simulink model "AM_signal"  (R2019b)
settings: Solver=VariableStepAuto  StartTime=0.0  StopTime=10.0  RelTol=1e-3
libraries: commchan3 x1, dspsnks4 x1, commanapbnd3 x1
settings Model: Creator=Kai  LastModifiedBy=Kai

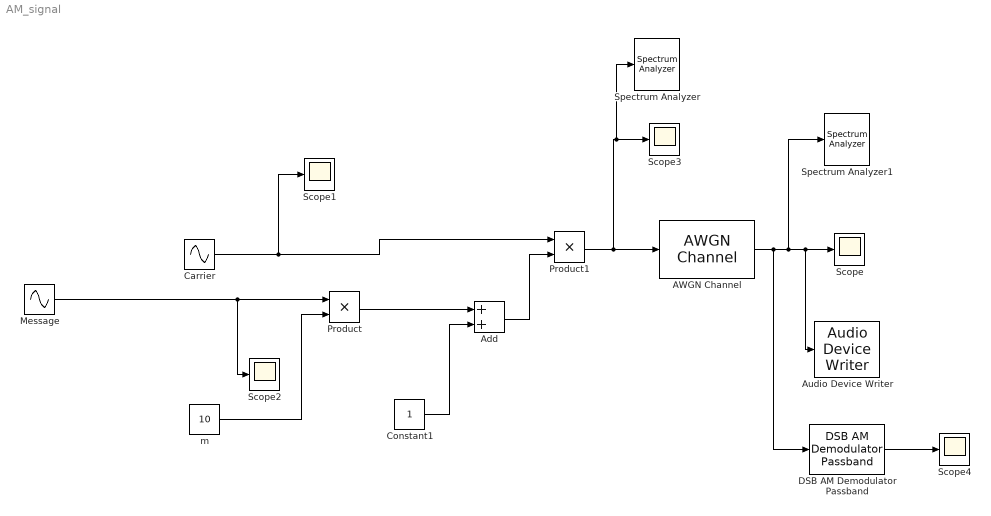
== system AM_signal ==
  AWGN Channel : commchan3/AWGN Channel  InputProcessing=Columns as channels (frame based)  seed=67  noiseMode="Signal to noise ratio  (SNR)"  EbNodB=10  EsNodB=10  SNRdB=3  bitsPerSym=1  Ps=1  Tsym=1  variance=1
      settings: SourceProductName=Communications Toolbox
  Add : Sum
  Audio Device Writer : dspsnks4/Audio Device Writer  Driver=DirectSound  Device=Default  InheritSampleRate=on  SampleRate=44100  BitDepth=16-bit integer  BufferSize=4096  NumBuffers=10  DefaultOutputChannelMapping=on  OutputChannelMapping=1:2  OutputNumUnderrunSamples=off  DriverIdx=1  DeviceWarnFlag=''
  Carrier : Sin  Frequency=2*pi*25  SampleTime=1/50000
  Constant1 : Constant
  DSB AM Demodulator Passband : commanapbnd3/DSB AM Demodulator Passband  Fc=300  Ph=0  method=Butterworth  n=4  cf=300  Rp=0.1  Rs=50  Offset=1
      settings: SourceProductName=Communications Toolbox  SourceProductBaseCode=CM
  "Message " : Sin  Frequency=2*pi  SampleTime=1/50000
  Product : Product
  Product1 : Product
  Scope{,1..4} (5 alike) : Scope
  Spectrum Analyzer : SpectrumAnalyzer
  Spectrum Analyzer1 : SpectrumAnalyzer
  m : Constant  Value=10
  wires:
  "Message "/1 -> Scope2/1, Product/1
  m/1 -> Product/2
  Carrier/1 -> Scope1/1, Product1/1
  Product/1 -> Add/1
  Constant1/1 -> Add/2
  Add/1 -> Product1/2
  AWGN Channel/1 -> DSB AM Demodulator Passband/1, Spectrum Analyzer1/1, Audio Device Writer/1, Scope/1
  Product1/1 -> Spectrum Analyzer/1, Scope3/1, AWGN Channel/1
  DSB AM Demodulator Passband/1 -> Scope4/1
